simulink model "City_Environment_TS2020"  (Simulink 8.1)
settings: Solver=ode45  StartTime=0.0  StopTime=25  RelTol=1e-3
libraries: Solver_SF x4
settings Model: Creator=elowe  LastModifiedBy=dreichenbach
settings DebuggingCC: FcnCallInpInsideContextMsg=EnableAllAsWarning  FrameProcessingCompatibilityMsg=error
settings GRTTargetCC: CodeReplacementLibrary=C89/C90 (ANSI)  CombineOutputUpdateFcns=on  GRTInterface=off

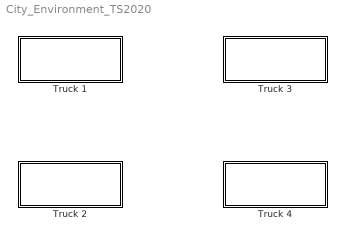
== system City_Environment_TS2020 ==
  Truck 1 : Subsystem
  Truck 2 : Subsystem
  Truck 3 : Subsystem
  Truck 4 : Subsystem

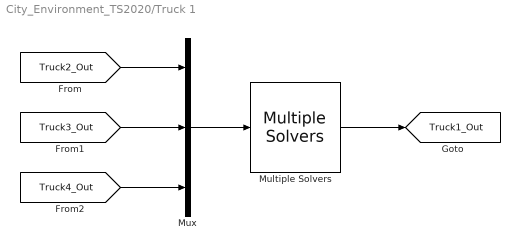
== system City_Environment_TS2020/Truck 1 ==
  Multiple Solvers : Solver_SF/Multiple Solvers  Priority=1  iVehicle=1  SIMFILE=D:\Product_Dev\trunk\Image\TruckSim\Core\TruckSim_Data\Extensions\Simulink\Multi_Vehicle\simfile1.sim  Run_RTs=off  vs_state_ind=Run  StopMode_ind=Vehicle Model  vs_scx=on
  Mux : Mux  Inputs=3
  tag scope: Truck1_Out=global
  wires:
  Mux/1 -> Multiple Solvers/1
  Multiple Solvers/1 -> [Truck1_Out]
  [Truck2_Out] -> Mux/1
  [Truck3_Out] -> Mux/2
  [Truck4_Out] -> Mux/3

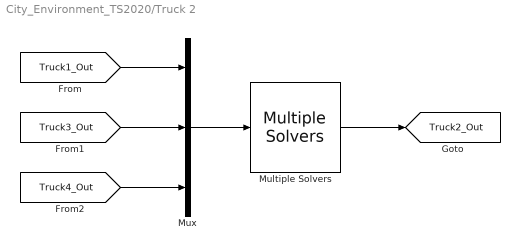
== system City_Environment_TS2020/Truck 2 ==
  Multiple Solvers : Solver_SF/Multiple Solvers  Priority=1  iVehicle=2  SIMFILE=D:\Product_Dev\trunk\Image\TruckSim\Core\TruckSim_Data\Extensions\Simulink\Multi_Vehicle\simfile2.sim  Run_RTs=off  vs_state_ind=Run  StopMode_ind=Vehicle Model  vs_scx=on
  Mux : Mux  Inputs=3
  tag scope: Truck2_Out=global
  wires:
  Mux/1 -> Multiple Solvers/1
  Multiple Solvers/1 -> [Truck2_Out]
  [Truck1_Out] -> Mux/1
  [Truck3_Out] -> Mux/2
  [Truck4_Out] -> Mux/3

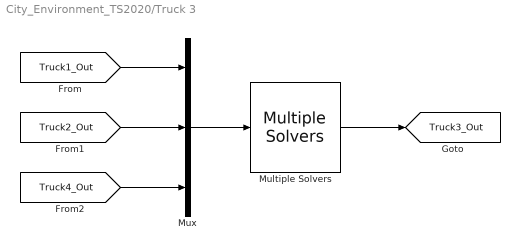
== system City_Environment_TS2020/Truck 3 ==
  Multiple Solvers : Solver_SF/Multiple Solvers  Priority=1  iVehicle=3  SIMFILE=D:\Product_Dev\trunk\Image\TruckSim\Core\TruckSim_Data\Extensions\Simulink\Multi_Vehicle\simfile3.sim  Run_RTs=off  vs_state_ind=Run  StopMode_ind=Vehicle Model  vs_scx=on
  Mux : Mux  Inputs=3
  tag scope: Truck3_Out=global
  wires:
  Mux/1 -> Multiple Solvers/1
  Multiple Solvers/1 -> [Truck3_Out]
  [Truck1_Out] -> Mux/1
  [Truck2_Out] -> Mux/2
  [Truck4_Out] -> Mux/3

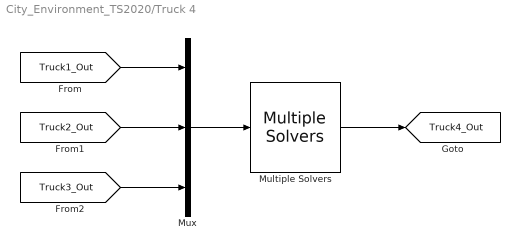
== system City_Environment_TS2020/Truck 4 ==
  Multiple Solvers : Solver_SF/Multiple Solvers  Priority=1  iVehicle=4  SIMFILE=D:\Product_Dev\trunk\Image\TruckSim\Core\TruckSim_Data\Extensions\Simulink\Multi_Vehicle\simfile4.sim  Run_RTs=off  vs_state_ind=Run  StopMode_ind=Vehicle Model  vs_scx=on
  Mux : Mux  Inputs=3
  tag scope: Truck4_Out=global
  wires:
  Mux/1 -> Multiple Solvers/1
  Multiple Solvers/1 -> [Truck4_Out]
  [Truck1_Out] -> Mux/1
  [Truck2_Out] -> Mux/2
  [Truck3_Out] -> Mux/3
